simulink model "OPC_AUTOMATIZACIO_PROCESOS"  (R2019a)
settings: Solver=ode45  StartTime=0.0  StopTime=inf  RelTol=1e-3  EnableMultiTasking=on
libraries: opclib x5
settings Model: Creator=user  LastModifiedBy=jvela
settings DataIOCC: LimitDataPoints=on  SaveFormat=Array  ReturnWorkspaceOutputs=off
settings OptimizationCC: LifeSpan=inf
settings DebuggingCC: SolverPrmCheckMsg=warning  SFUnexpectedBacktrackingDiag=warning  SFNoUnconditionalDefaultTransitionDiag=warning  SFExecutionAtInitializationDiag=none  ArithmeticOperatorsInVariantConditions=warning
settings HardwareCC: ProdBitPerPointer=32  ProdBitPerSizeT=32  ProdBitPerPtrDiffT=32  ProdLargestAtomicFloat=None  ProdIntDivRoundTo=Undefined  ProdEndianess=Unspecified  ProdWordSize=32  ProdHWDeviceType=32-bit Generic
settings ModelReferenceCC: PropagateSignalLabelsOutOfModel=off
settings SFSimCC: SimUseLocalCustomCode=off
settings RTWCC: RTWUseLocalCustomCode=off
settings CodeAppCC: StateflowObjectComments=on
settings GRTTargetCC: TargetLangStandard=C89/C90 (ANSI)  GeneratePreprocessorConditionals=Disable all
settings ConfigComp: CovMetricSettings=dw  CovHtmlReporting=on  CovSaveCumulativeToWorkspaceVar=on  CovSaveSingleToWorkspaceVar=on  CovExternalEMLEnable=off  CovSFcnEnable=off

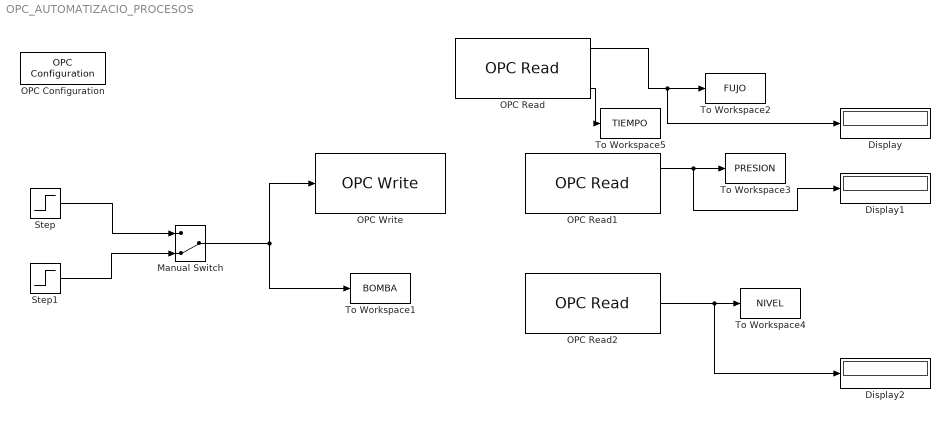
== system OPC_AUTOMATIZACIO_PROCESOS ==
  Display : Display
  Display1 : Display
  Display2 : Display
  Manual Switch : ManualSwitch  CurrentSetting=0
  OPC Configuration : opclib/OPC Configuration  opcServers=localhost/Kepware.KEPServerEX.V6/10  errMissingItems=Error  errReadWrite=Warn  errShutdown=Error  errRTViolation=Warn  rtEnable=on  speedup=1  showLatency=off  beingUsed=on
      settings: SourceProductName=OPC Toolbox  SourceProductBaseCode=OT
  OPC Read : opclib/OPC Read  serverHost=localhost  serverID=Kepware.KEPServerEX.V6  itemIDs=1500.Device1.FLUJO  readMode=Synchronous (cache)  dataType=double  updateRate=0.5  showQual=on  showTS=on  tsMode=Seconds since start
      settings: SourceProductName=OPC Toolbox  SourceProductBaseCode=OT
  OPC Read1 : opclib/OPC Read  serverHost=localhost  serverID=Kepware.KEPServerEX.V6  itemIDs=1500.Device1.PRESION  readMode=Synchronous (cache)  dataType=double  updateRate=0.5  showQual=off  showTS=on  tsMode=Seconds since start
      settings: SourceProductName=OPC Toolbox  SourceProductBaseCode=OT
  OPC Read2 : opclib/OPC Read  serverHost=localhost  serverID=Kepware.KEPServerEX.V6  itemIDs=1500.Device1.NIVEL  readMode=Synchronous (cache)  dataType=double  updateRate=0.5  showQual=off  showTS=off  tsMode=Seconds since start
      settings: SourceProductName=OPC Toolbox  SourceProductBaseCode=OT
  OPC Write : opclib/OPC Write  serverHost=localhost  serverID=Kepware.KEPServerEX.V6  itemIDs=1500.Device1.BOMBA  writeMode=Synchronous  updateRate=0.5
      settings: SourceProductName=OPC Toolbox  SourceProductBaseCode=OT
  Step : Step  Time=0  After=27000  SampleTime=0.5
  Step1 : Step  Time=0  After=0  SampleTime=0.5
  To Workspace1 : ToWorkspace  VariableName=BOMBA  SampleTime=-1
  To Workspace2 : ToWorkspace  VariableName=FUJO  SampleTime=-1
  To Workspace3 : ToWorkspace  VariableName=PRESION  SampleTime=-1
  To Workspace4 : ToWorkspace  VariableName=NIVEL  SampleTime=-1
  To Workspace5 : ToWorkspace  VariableName=TIEMPO  SampleTime=-1
  wires:
  Manual Switch/1 -> OPC Write/1, To Workspace1/1
  Step/1 -> Manual Switch/1
  Step1/1 -> Manual Switch/2
  OPC Read/1 -> Display/1, To Workspace2/1
  OPC Read1/1 -> Display1/1, To Workspace3/1
  OPC Read2/1 -> Display2/1, To Workspace4/1
  OPC Read/3 -> To Workspace5/1
